simulink subsystem "Control_Selector"  (R2024a)
settings: Solver=VariableStepAuto  StartTime=0.0  StopTime=10.0  RelTol=1e-3
settings Model: Creator=gurt1  LastModifiedBy=gurt1

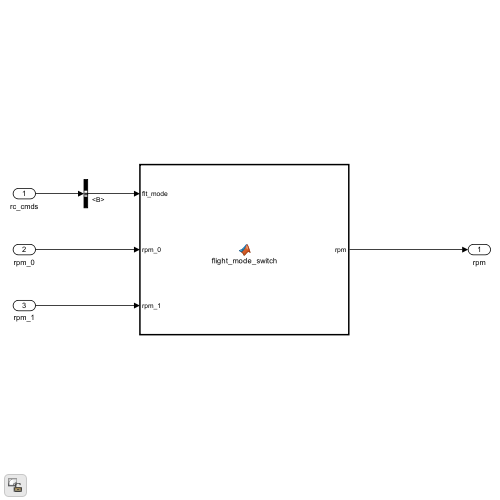
[thumbnail: Simulink's stored preview of the top-level diagram]
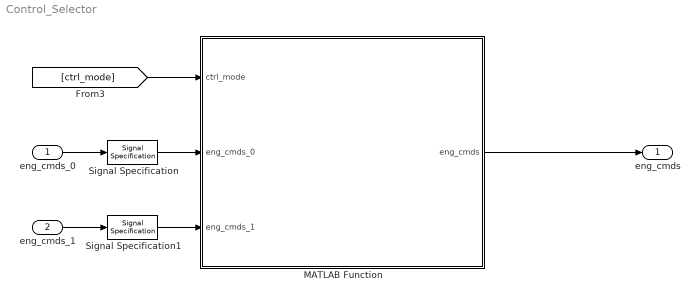
== system Control_Selector ==
  eng_cmds_0 : Inport
  eng_cmds_1 : Inport  Port=2
  MATLAB Function : MATLAB Function  TreatAsAtomicUnit=on
  Signal Specification : SignalSpecification  Dimensions=16
  Signal Specification1 : SignalSpecification  Dimensions=16
  eng_cmds : Outport
  wires:
  eng_cmds_0/1 -> Signal Specification/1
  eng_cmds_1/1 -> Signal Specification1/1
  MATLAB Function/1(eng_cmds) -> eng_cmds/1
  [ctrl_mode] -> MATLAB Function/1(ctrl_mode)
  Signal Specification/1 -> MATLAB Function/2(eng_cmds_0)
  Signal Specification1/1 -> MATLAB Function/3(eng_cmds_1)

== matlab function Control_Selector/MATLAB Function ==
  data: ctrl_mode input; eng_cmds output; eng_cmds_0 input; eng_cmds_1 input
% This function selects between two different sets of engineering commands and
% outputs the proper one dependant on control mode selection

function eng_cmds = flight_mode_switch(ctrl_mode, eng_cmds_0, eng_cmds_1)
    if ctrl_mode >= 0.5
        eng_cmds = eng_cmds_1;
    else
        eng_cmds = eng_cmds_0;
    end
end
